simulink model "FIR_Asymmetric_Decimation_Ex2"  (R2024a)
settings: Solver=VariableStepAuto  StartTime=0.0  StopTime=1  RelTol=1e-3
PostLoadFcn:
  | % All frequency values are in Hz.
  | Fs = 100000;  % Sampling Frequency
  | Fpass = 5000;              % Passband Frequency
  | Fstop = 10000;             % Stopband Frequency
  | Dpass = 0.0046051376314;   % Passband Ripple
  | Dstop = 0.00025118864315;  % Stopband Attenuation
  | dens  = 16;                % Density Factor
  | % Calculate the order from the parameters using FIRPMORD.
  | [N, Fo, Ao, W] = firpmord([Fpass, Fstop]/(Fs/2), [1 0], [Dpass, Dstop]);
  | % Calculate the coefficients using the FIRPM function.
  | coeffs = firpm(N, Fo, Ao, W, {dens});
  | % Hd = dsp.FIRFilter( ...
  | %     'Numerator', b);
undefined symbols (not defined in the file): designMultirateFIR, None, S, vsva2197, xcvc1902
libraries: dspsrcs4 x1, aieDSP x1, dspmlti4 x1, vmcUtilities x1
settings Model: Creator=sdegala  LastModifiedBy=robg
settings ModelReferenceCC: EnableRefExpFcnMdlSchedulingChecks=on
settings RTWCC: GPUComputeCapability=3.5
settings ConfigComp: CovBoundaryAbsTol=1.0e-5

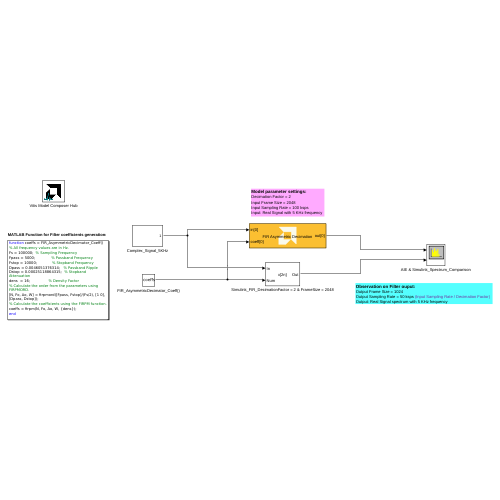
[thumbnail: Simulink's stored preview of the top-level diagram]
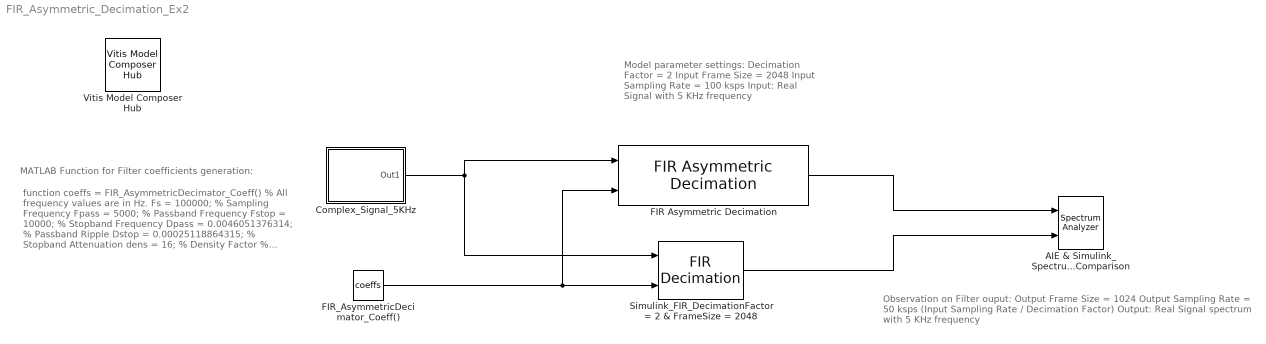
== system FIR_Asymmetric_Decimation_Ex2 ==
  note: Observation on Filter ouput:
      | Output Frame Size = 1024
      | Output Sampling Rate = 50 ksps (Input Sampling Rate / Decimation Factor)
      | Output: Real Signal spectrum with 5 KHz frequency
  note: Model parameter settings:
      | Decimation Factor = 2
      | Input Frame Size = 2048
      | Input Sampling Rate = 100 ksps
      | Input: Real Signal with 5 KHz frequency
  note: MATLAB Function for Filter coefficients generation:
  note: function coeffs = FIR_AsymmetricDecimator_Coeff()
      | % All frequency values are in Hz.
      | Fs = 100000; % Sampling Frequency
      | Fpass = 5000; % Passband Frequency
      | Fstop = 10000; % Stopband Frequency
      | Dpass = 0.0046051376314; % Passband Ripple
      | Dstop = 0.00025118864315; % Stopband Attenuation
      | dens = 16; % Density Factor
      | % Calculate the order from the parameters using FIRPMORD.
      | [N, Fo, Ao, W] = firpmord([Fpass, Fstop]/(Fs/2), [1 0], [Dpass, Dstop]);
      | % Calculate the coefficients using the FIRPM function.
      | coeffs = firpm(N, Fo, Ao, W, {dens});
      | end
  AIE & Simulink_Spectrum_Comparison : SpectrumAnalyzer  NumInputPorts=2  AveragingMethod=Exponential  ChannelNames="[\"\"]"  AllowFFTLengthLessThanSamplesPerUpdate=on  DefaultConfigurationName=spbscopes.SpectrumAnalyzerBlockCfg
  Complex_Signal_5KHz : Subsystem
  FIR Asymmetric Decimation : aieDSP/FIR Asymmetric Decimation  data_type=float  coef_type=float  use_coeff_reload=on  num_outputs=off  coeff=[1, zeros(1,31)]  fir_length=64  decimate_factor=2  input_window_size=2048  shift_val=0  rnd_mode=Round to positive infinity  sat_mode=0-None  deci_poly=1  casc_length=1  AIE_VARIANT=1  dual_ip=0  TP_API=0  ssr=1  blockJsonConstraints=[]  blockJsonConstraintsInternal=[]  spec=vmc_fir_decimate_asym.json  SerializedMaskParamNames=[]  SerializedMaskParamValues=[]  SerializedMaskParamVisibilities=[]  block_type=FIR Asymmetric Decimation  SerializedMaskParamDataypes=typename|typename|uint|uint|coef_type|uint|uint|uint|uint|uint|uint|uint|uint|uint|uint|uint|uint  SerializedMaskParamEnumStrArr=0|0|0|0|0|0|0|0|0|Floor,Ceiling,Round to positive infinity,Round to negative infinity,Round symmetrical to infinity,Round symmetrical to zero,Round convergent to even,Round convergent to odd|0-None,1-Asymmetric,3-Symmetric|0|0|0|0|0|0  SerializedMaskParamEnumValArr=0|0|0|0|0|0|0|0|0|0,1,2,3,4,5,6,7|0,1,3|0|0|0|0|0|0  SerializedMaskParamVectorArr=0|0|0|0|1|0|0|0|0|0|0|0|0|0|0|0|0  SerializedMaskParamKeys=TT_DATA|TT_COEFF|TP_USE_COEFF_RELOAD|TP_NUM_OUTPUTS|coeff|TP_FIR_LEN|TP_DECIMATE_FACTOR|TP_INPUT_WINDOW_VSIZE|TP_SHIFT|TP_RND|TP_SAT|TP_PARA_DECI_POLY|TP_CASC_LEN|AIE_VARIANT|TP_DUAL_IP|TP_API|TP_SSR
  FIR_AsymmetricDecimator_Coeff() : Constant  Value=coeffs  OutDataTypeStr=single
  Simulink_FIR_DecimationFactor = 2 & FrameSize = 2048 : dspmlti4/FIR Decimation  FilterSource=Input port  h=designMultirateFIR(1,2)  D=2  filtStruct=Direct form  FilterObject=FDECIM  InputProcessing=Columns as channels (frame based)  framing=Enforce single-rate processing  AllowArbitraryInputLength=off  inputOffset=0  outputBufInitCond=0  roundingMode=Floor  overflowMode=off  firstCoeffDataTypeStr=Inherit: Same word length as input  firstCoeffMin=[]  firstCoeffMax=[]  firstCoeffLastDataTypeStr=Inherit: Same word length as input  outputDataTypeStr=Inherit: Same as accumulator  outputMin=[]  outputMax=[]  outputLastDataTypeStr=Inherit: Same as accumulator
  Vitis Model Composer Hub : vmcUtilities/Vitis Model Composer Hub  Tag=genX  CodeGeneration=off  StartColumn=1  NumberOfColumns=1  TargetDirectory=./code  exportDesign=off  analyzeDesign=off  validateDesignOnHw=off  ExportType=AI Engines  IpVendor=xilinx.com  IpLibrary=hls  IpVersion=1.0  IpHWLanguage=Verilog  AieCompilerOptions={}  AieSimulatorOptions={}  CreateTestbench=off  TestbenchStackSize=10  RunRtlSim=off  RunCSim=off  RunAieSim=off  AieSimTimeout=50000  RunAieSimProfiling=off  LaunchVitisAnalyzer=off  PlotOutput=off  RunX86Sim=off  X86SimTimeout=10  GenHwImage=off  GenLibadfXo=off  GenHwValidationCode=off  PlatformType=Not Specified  HwSystemType=Baremetal  HwValidationTarget=hw  ProjDevice=xcvc1902-vsva2197-1LP-e-S  ProjDevicePart=xcvc1902-vsva2197-1LP-e-S  AIEType=AIE  SamplePeriod=-1  ClockFrequency=200  DataPathParallelism=1  xilinxfamily=versalaicore  part=xcvc1902  speed=-1LP-e-S  package=vsva2197  directory=./netlist  testbench=off  incr_netlist=off  synthesis_tool=Vivado  clock_wrapper=Clock Enables  dbl_ovrd=According to Block Masks  dcm_input_clock_period=10  sysclk_period=10  simulink_period=1  eval_field=0  LogFileName=''  NThreads=4
  wires:
  FIR_AsymmetricDecimator_Coeff()/1 -> FIR Asymmetric Decimation/2, Simulink_FIR_DecimationFactor = 2 & FrameSize = 2048/2
  Complex_Signal_5KHz/1(Out1) -> FIR Asymmetric Decimation/1, Simulink_FIR_DecimationFactor = 2 & FrameSize = 2048/1
  FIR Asymmetric Decimation/1 -> AIE & Simulink_Spectrum_Comparison/1
  Simulink_FIR_DecimationFactor = 2 & FrameSize = 2048/1 -> AIE & Simulink_Spectrum_Comparison/2

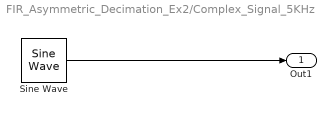
== system FIR_Asymmetric_Decimation_Ex2/Complex_Signal_5KHz ==
  Sine Wave : dspsrcs4/Sine Wave  Amplitude=1  Frequency=5e3  Phase=0  SampleMode=Discrete  OutComplex=Real  CompMethod=Trigonometric fcn  TableSize=Speed  SampleTime=1/100e3  SamplesPerFrame=2048  ResetState=Restart at time zero  OutputFrames=off  dataType=single  wordLen=16  udDataType=sfix(16)  fracBitsMode=Best precision  numFracBits=15  OutDataTypeStr=single  LastOutDataTypeStr=single
  Out1 : Outport
  wires:
  Sine Wave/1 -> Out1/1
